simulink model "ControlSim"  (R2020b)
settings: Solver=VariableStepAuto  StartTime=0.0  StopTime=T  RelTol=1e-3
values from neighbouring files (symbols this model uses):
  condtheta = x0(3)    [MPCdefinition.m]
  condx = x0(1)    [MPCdefinition.m]
  condy = x0(2)    [MPCdefinition.m]
  dim_platform = 1.3    [MPCdefinition.m]
  k_obsx = 5    [MPCdefinition.m]
  k_obsy = 5    [MPCdefinition.m]
  omega_max_perc = 0.1    [MPCdefinition.m]
  omega_min_perc = -0.1    [MPCdefinition.m]
  omega_sat = 2    [MPCdefinition.m]
  slope_circ = 0.2    [MPCdefinition.m]
  v_max_perc = 0.5    [MPCdefinition.m]
  v_min_perc = -0.5    [MPCdefinition.m]
  v_square = 0.8    [MPCdefinition.m]
libraries: simulink x3, mpclib x1
settings Model: Creator=adelina  LastModifiedBy=adelina

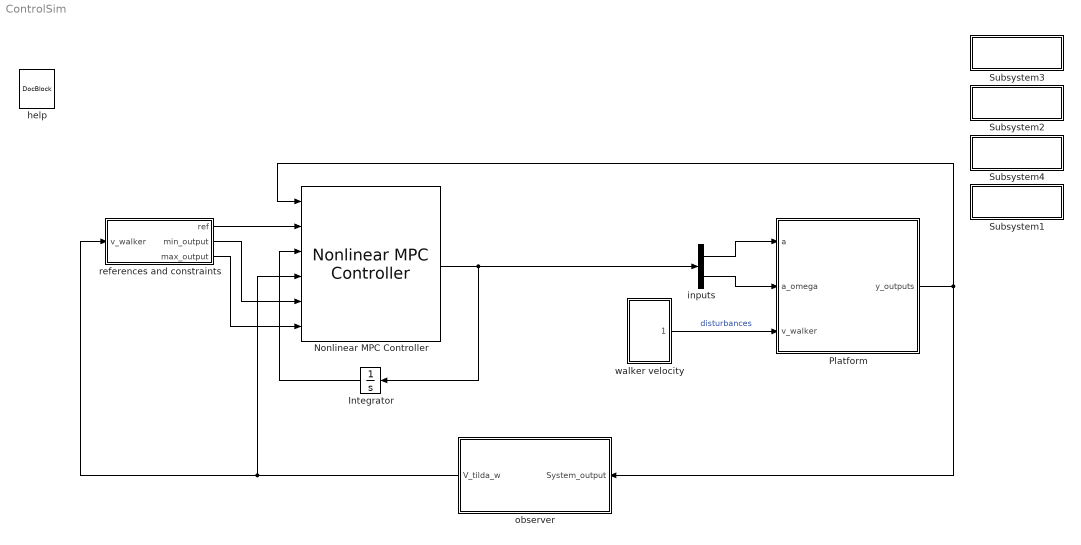
== system ControlSim ==
  Integrator : Integrator  InitialCondition=[0, 0]
  Nonlinear MPC Controller : mpclib/Nonlinear MPC Controller  SCDEnableBlockLinearizationSpecification=on  nlmpcobj=nlobj  UseObjectTs=on  UseMEX=off  md_enabled=on  mvtarget_enabled=off  param_enabled=off  cost_enabled=off  mvseq_enabled=off  stateseq_enabled=off  ovseq_enabled=off  slack_enabled=off  status_enabled=off  ov_min=on  ov_max=on  mv_min=off  mv_max=off  mvrate_min=off  mvrate_max=off  state_min=off  state_max=off  ov_weight=off  mv_weight=off  mvrate_weight=off  ecr_weight=off  nlp_initialize=off
  Platform : Subsystem
  Subsystem1 : Subsystem
      settings: OpenFcn=animation
      mask Display: disp('Animation')
  Subsystem2 : Subsystem
      settings: OpenFcn=plot_inputs
      mask Display: disp('plot inputs')
  Subsystem3 : Subsystem
      settings: OpenFcn=plot_states
      mask Display: disp('plot states')
  Subsystem4 : Subsystem
      settings: OpenFcn=plot_trajectory_frames
      mask Display: disp('plot trajectory')
  help : simulink/Model-Wide Utilities/DocBlock  DocumentType=Text
      content=|
      | 1. You may have errors running plot trajectory, this is due to the "for ... end" in the script, just ignore the error
      |
      | 2. To choose the trajectory go on the block "walker velocity"
  inputs : Demux  Outputs=2
  observer : Subsystem
  references and constraints : Subsystem
  walker velocity : Subsystem
  wires:
  inputs/2 -> Platform/2(a_omega)
  inputs/1 -> Platform/1(a)
  Integrator/1 -> Nonlinear MPC Controller/3
  references and constraints/1(ref) -> Nonlinear MPC Controller/2
  Platform/1(y_outputs) -> observer/1(System_output), Nonlinear MPC Controller/1
  walker velocity/1(v_walker) -> Platform/3(v_walker)  "disturbances"
  observer/1(V_tilda_w) -> Nonlinear MPC Controller/4, references and constraints/1(v_walker)
  references and constraints/2(min_output) -> Nonlinear MPC Controller/5
  references and constraints/3(max_output) -> Nonlinear MPC Controller/6
  Nonlinear MPC Controller/1 -> inputs/1, Integrator/1

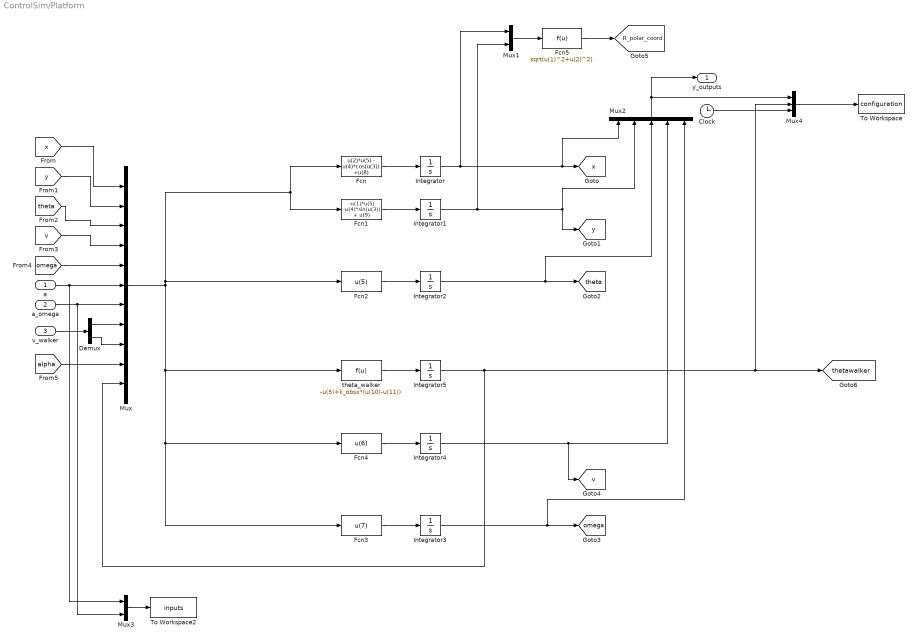
== system ControlSim/Platform ==
  a : Inport
  a_omega : Inport  Port=2
  v_walker : Inport  Port=3
  Clock : Clock
  Demux : Demux  Outputs=2
  Fcn : Fcn  Expr=u(2)*u(5) - u(4)*cos(u(3)) +u(8)
  Fcn1 : Fcn  Expr=-u(1)*u(5) -u(4)*sin(u(3)) + u(9)
  Fcn2 : Fcn  Expr=u(5)
  Fcn3 : Fcn  Expr=u(7)
  Fcn4 : Fcn  Expr=u(6)
  Fcn5 : Fcn  Expr=sqrt(u(1)^2+u(2)^2)
  Integrator : Integrator  InitialCondition=condx
  Integrator1 : Integrator  InitialCondition=condy
  Integrator2 : Integrator  InitialCondition=condtheta
  Integrator3 : Integrator
  Integrator4 : Integrator
  Integrator5 : Integrator  InitialCondition=condtheta
  Mux : Mux  Inputs=11
  Mux1 : Mux  Inputs=2
  Mux2 : Mux  Inputs=5
  Mux3 : Mux  Inputs=2
  Mux4 : Mux  Inputs=3
  To Workspace : ToWorkspace  VariableName=configuration  SaveFormat=Structure With Time  SampleTime=-1
  To Workspace2 : ToWorkspace  VariableName=inputs  SaveFormat=Structure With Time  SampleTime=-1
  theta_walker : Fcn  Expr=-u(5)+k_obsx*(u(10)-u(11))
  y_outputs : Outport
  tag scope: R_polar_coord=global, omega=global, theta=global, thetawalker=global, v=global, x=global, y=global
  wires:
  Fcn2/1 -> Integrator2/1
  Integrator2/1 -> [theta], Mux2/3
  Fcn1/1 -> Integrator1/1
  [y] -> Mux/2
  [x] -> Mux/1
  a/1 -> Mux3/1, Mux/6
  Integrator1/1 -> Mux1/2, [y], Mux2/2
  [theta] -> Mux/3
  Integrator/1 -> Mux1/1, Mux2/1, [x]
  Fcn/1 -> Integrator/1
  a_omega/1 -> Mux3/2, Mux/7
  Mux2/1 -> y_outputs/1, Mux4/1
  [v] -> Mux/4
  [omega] -> Mux/5
  Integrator3/1 -> Mux2/5, [omega]
  Fcn3/1 -> Integrator3/1
  Integrator4/1 -> [v], Mux2/4
  Fcn4/1 -> Integrator4/1
  Mux1/1 -> Fcn5/1
  Fcn5/1 -> [R_polar_coord]
  Mux3/1 -> To Workspace2/1
  Clock/1 -> Mux4/3
  Mux4/1 -> To Workspace/1
  v_walker/1 -> Demux/1
  Demux/1 -> Mux/8
  Demux/2 -> Mux/9
  [alpha] -> Mux/10
  Mux/1 -> Fcn1/1, Fcn/1, Fcn2/1, theta_walker/1, Fcn3/1, Fcn4/1
  theta_walker/1 -> Integrator5/1
  Integrator5/1 -> Mux/11, [thetawalker], Mux4/2

== system ControlSim/Subsystem1 ==

== system ControlSim/Subsystem2 ==

== system ControlSim/Subsystem3 ==

== system ControlSim/Subsystem4 ==

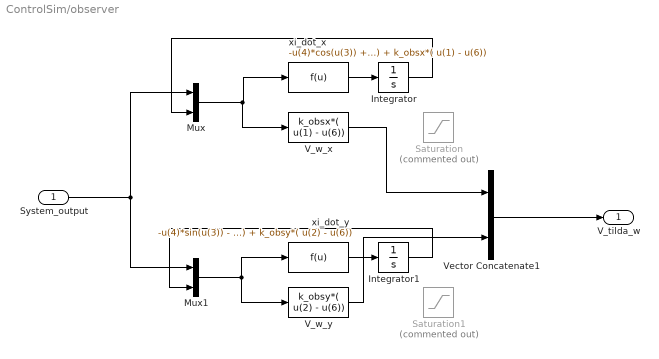
== system ControlSim/observer ==
  System_output : Inport
  Integrator : Integrator  InitialCondition=condx
  Integrator1 : Integrator  InitialCondition=condy
  Mux : Mux  Inputs=2
  Mux1 : Mux  Inputs=2
  Saturation : Saturate  Commented=on
  Saturation1 : Saturate  Commented=on
  V_w_x : Fcn  Expr=k_obsx*( u(1) - u(6))
  V_w_y : Fcn  Expr=k_obsy*( u(2) - u(6))
  Vector Concatenate1 : Concatenate  Mode=Multidimensional array  ConcatenateDimension=2
  xi_dot_x : Fcn  Expr=-u(4)*cos(u(3)) + u(2)*u(5) + k_obsx*( u(1) - u(6))
  xi_dot_y : Fcn  Expr=-u(4)*sin(u(3)) - u(1)*u(5) + k_obsy*( u(2) - u(6))
  V_tilda_w : Outport
  wires:
  Mux/1 -> V_w_x/1, xi_dot_x/1
  Mux1/1 -> V_w_y/1, xi_dot_y/1
  System_output/1 -> Mux/1, Mux1/1
  Vector Concatenate1/1 -> V_tilda_w/1
  xi_dot_x/1 -> Integrator/1
  Integrator/1 -> Mux/2
  xi_dot_y/1 -> Integrator1/1
  Integrator1/1 -> Mux1/2
  V_w_y/1 -> Vector Concatenate1/2
  V_w_x/1 -> Vector Concatenate1/1

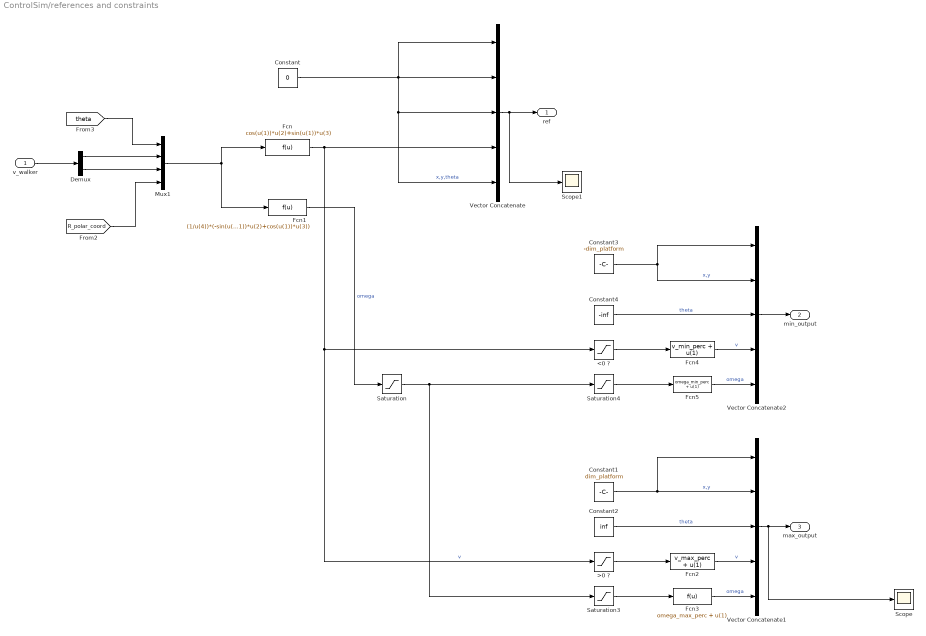
== system ControlSim/references and constraints ==
  v_walker : Inport
  <0 ? : Saturate  UpperLimit=0  LowerLimit=-inf
  >0 ? : Saturate  UpperLimit=inf  LowerLimit=0
  Constant : Constant  Value=0
  Constant1 : Constant  Value=dim_platform
  Constant2 : Constant  Value=inf
  Constant3 : Constant  Value=-dim_platform
  Constant4 : Constant  Value=-inf
  Demux : Demux  Outputs=2
  Fcn : Fcn  Expr=cos(u(1))*u(2)+sin(u(1))*u(3)
  Fcn1 : Fcn  Expr=(1/u(4))*(-sin(u(1))*u(2)+cos(u(1))*u(3))
  Fcn2 : Fcn  Expr=v_max_perc + u(1)
  Fcn3 : Fcn  Expr=omega_max_perc + u(1)
  Fcn4 : Fcn  Expr=v_min_perc + u(1)
  Fcn5 : Fcn  Expr=omega_min_perc + u(1)
  Mux1 : Mux
  Saturation : Saturate  UpperLimit=omega_sat  LowerLimit=-omega_sat
  Saturation3 : Saturate  UpperLimit=inf  LowerLimit=0
  Saturation4 : Saturate  UpperLimit=0  LowerLimit=-inf
  Scope : Scope
  Scope1 : Scope
  Vector Concatenate : Concatenate  NumInputs=5  Mode=Multidimensional array  ConcatenateDimension=2
  Vector Concatenate1 : Concatenate  NumInputs=5  Mode=Multidimensional array  ConcatenateDimension=2
  Vector Concatenate2 : Concatenate  NumInputs=5  Mode=Multidimensional array  ConcatenateDimension=2
  ref : Outport
  min_output : Outport  Port=2
  max_output : Outport  Port=3
  wires:
  Constant/1 -> Vector Concatenate/1, Vector Concatenate/5, Vector Concatenate/3, Vector Concatenate/2  "x,y,theta"
  Vector Concatenate/1 -> Scope1/1, ref/1
  [R_polar_coord] -> Mux1/4
  [theta] -> Mux1/1
  Demux/1 -> Mux1/2
  Demux/2 -> Mux1/3
  Fcn1/1 -> Saturation/1  "omega"
  Fcn2/1 -> Vector Concatenate1/4  "v"
  Constant1/1 -> Vector Concatenate1/1, Vector Concatenate1/2  "x,y"
  Mux1/1 -> Fcn/1, Fcn1/1
  Fcn3/1 -> Vector Concatenate1/5  "omega"
  Constant2/1 -> Vector Concatenate1/3  "theta"
  >0 ?/1 -> Fcn2/1
  Saturation3/1 -> Fcn3/1
  Fcn5/1 -> Vector Concatenate2/5  "omega"
  Constant4/1 -> Vector Concatenate2/3  "theta"
  Saturation/1 -> Saturation3/1, Saturation4/1
  Fcn/1 -> Vector Concatenate/4, >0 ?/1, <0 ?/1  "v"
  Fcn4/1 -> Vector Concatenate2/4  "v"
  Saturation4/1 -> Fcn5/1
  <0 ?/1 -> Fcn4/1
  Constant3/1 -> Vector Concatenate2/2, Vector Concatenate2/1  "x,y"
  Vector Concatenate2/1 -> min_output/1
  Vector Concatenate1/1 -> Scope/1, max_output/1
  v_walker/1 -> Demux/1

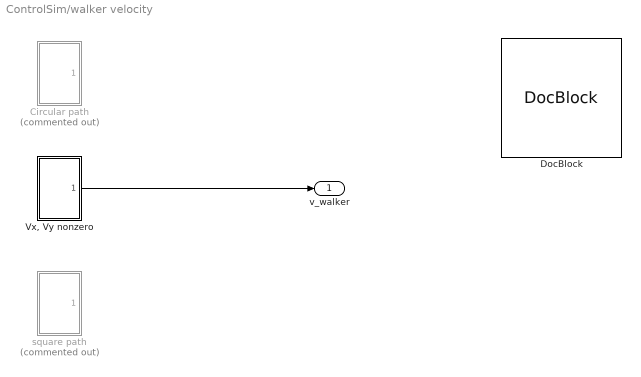
== system ControlSim/walker velocity ==
  Circular path : Subsystem  Commented=on
  DocBlock : simulink/Model-Wide Utilities/DocBlock  DocumentType=Text
      content=|
      | Choose one of the trajectory by uncommenting and connecting with the output
  "Vx, Vy nonzero" : Subsystem
  square path : Subsystem  Commented=on
  v_walker : Outport
  wires:
  "Vx, Vy nonzero"/1(v_walker) -> v_walker/1

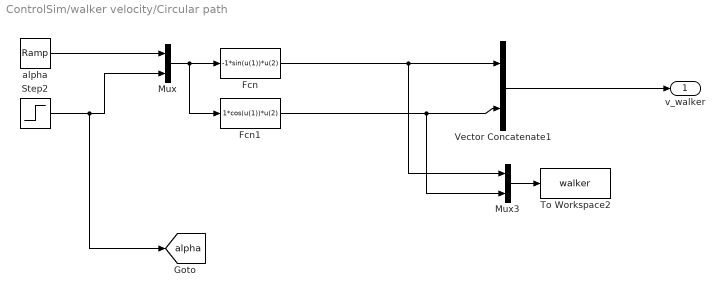
== system ControlSim/walker velocity/Circular path ==
  Fcn : Fcn  Expr=-1*sin(u(1))*u(2)
  Fcn1 : Fcn  Expr=1*cos(u(1))*u(2)
  Mux : Mux  Inputs=2
  Mux3 : Mux  Inputs=2
  Step2 : Step  After=slope_circ  SampleTime=0
  To Workspace2 : ToWorkspace  VariableName=walker  SaveFormat=Structure With Time  SampleTime=-1
  Vector Concatenate1 : Concatenate  Mode=Multidimensional array  ConcatenateDimension=2
  alpha : simulink/Sources/Ramp  slope=slope_circ  start=1  InitialOutput=0
  v_walker : Outport
  tag scope: alpha=global
  wires:
  alpha/1 -> Mux/1
  Fcn1/1 -> Vector Concatenate1/2, Mux3/2
  Fcn/1 -> Mux3/1, Vector Concatenate1/1
  Vector Concatenate1/1 -> v_walker/1
  Mux3/1 -> To Workspace2/1
  Mux/1 -> Fcn1/1, Fcn/1
  Step2/1 -> [alpha], Mux/2

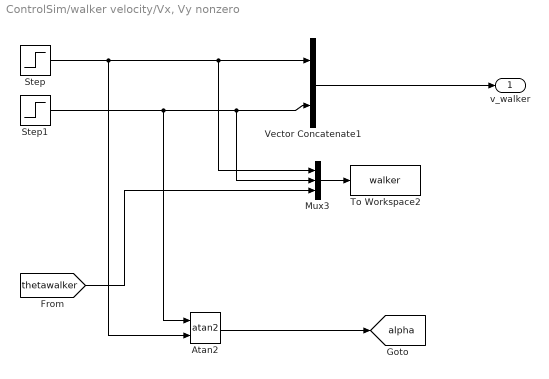
== system ControlSim/walker velocity/Vx, Vy nonzero ==
  Atan2 : Trigonometry  Operator=atan2
  Mux3 : Mux  Inputs=3
  Step : Step  Time=12  After=0.7  SampleTime=0
  Step1 : Step  Time=2  After=0.4  SampleTime=0
  To Workspace2 : ToWorkspace  VariableName=walker  SaveFormat=Structure With Time  SampleTime=-1
  Vector Concatenate1 : Concatenate  Mode=Multidimensional array  ConcatenateDimension=2
  v_walker : Outport
  tag scope: alpha=global
  wires:
  Vector Concatenate1/1 -> v_walker/1
  Mux3/1 -> To Workspace2/1
  Step/1 -> Atan2/2, Mux3/1, Vector Concatenate1/1
  Step1/1 -> Atan2/1, Vector Concatenate1/2, Mux3/2
  [thetawalker] -> Mux3/3
  Atan2/1 -> [alpha]

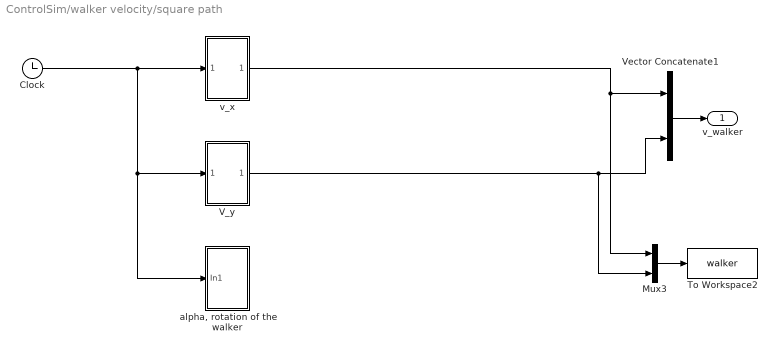
== system ControlSim/walker velocity/square path ==
  Clock : Clock
  Mux3 : Mux  Inputs=2
  To Workspace2 : ToWorkspace  VariableName=walker  SaveFormat=Structure With Time  SampleTime=-1
  V_y : Subsystem
  Vector Concatenate1 : Concatenate  Mode=Multidimensional array  ConcatenateDimension=2
  "alpha, rotation of the walker" : Subsystem
  v_x : Subsystem
  v_walker : Outport
  wires:
  Vector Concatenate1/1 -> v_walker/1
  Mux3/1 -> To Workspace2/1
  Clock/1 -> v_x/1(In1), "alpha, rotation of the walker"/1(In1), V_y/1(In1)
  V_y/1(Out1) -> Mux3/2, Vector Concatenate1/2
  v_x/1(Out1) -> Mux3/1, Vector Concatenate1/1

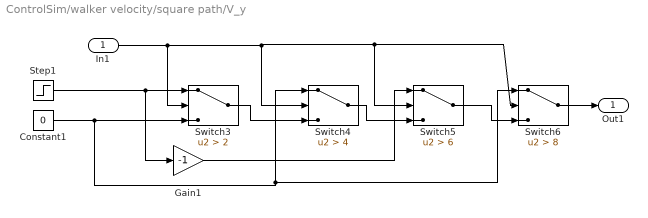
== system ControlSim/walker velocity/square path/V_y ==
  In1 : Inport
  Constant1 : Constant  Value=0
  Gain1 : Gain  Gain=-1
  Step1 : Step  Time=0  After=v_square  SampleTime=0
  Switch3 : Switch  Criteria=u2 > Threshold  Threshold=2
  Switch4 : Switch  Criteria=u2 > Threshold  Threshold=4
  Switch5 : Switch  Criteria=u2 > Threshold  Threshold=6
  Switch6 : Switch  Criteria=u2 > Threshold  Threshold=8
  Out1 : Outport
  wires:
  Step1/1 -> Gain1/1, Switch3/1
  Switch6/1 -> Out1/1
  In1/1 -> Switch3/2, Switch5/2, Switch6/2, Switch4/2
  Switch5/1 -> Switch6/3
  Switch3/1 -> Switch4/3
  Constant1/1 -> Switch6/1, Switch4/1, Switch3/3
  Switch4/1 -> Switch5/3
  Gain1/1 -> Switch5/1

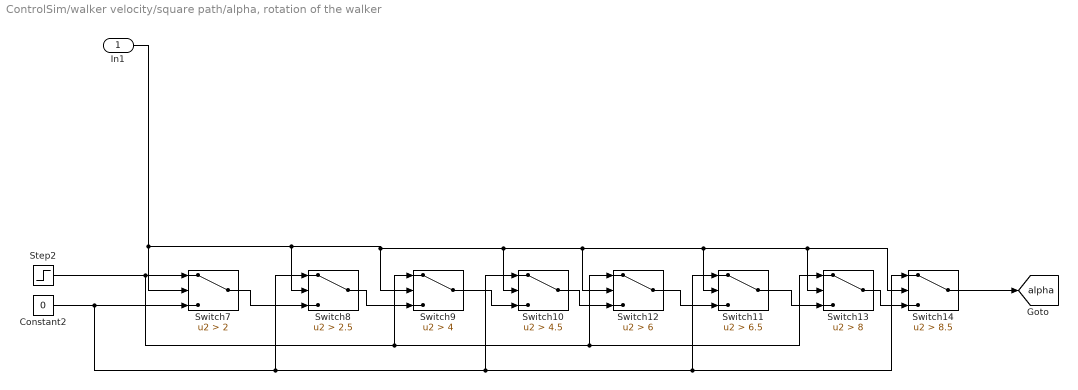
== system ControlSim/walker velocity/square path/alpha, rotation of the walker ==
  In1 : Inport
  Constant2 : Constant  Value=0
  Step2 : Step  Time=0  After=pi  SampleTime=0
  Switch10 : Switch  Criteria=u2 > Threshold  Threshold=4.5
  Switch11 : Switch  Criteria=u2 > Threshold  Threshold=6.5
  Switch12 : Switch  Criteria=u2 > Threshold  Threshold=6
  Switch13 : Switch  Criteria=u2 > Threshold  Threshold=8
  Switch14 : Switch  Criteria=u2 > Threshold  Threshold=8.5
  Switch7 : Switch  Criteria=u2 > Threshold  Threshold=2
  Switch8 : Switch  Criteria=u2 > Threshold  Threshold=2.5
  Switch9 : Switch  Criteria=u2 > Threshold  Threshold=4
  tag scope: alpha=global
  wires:
  Switch11/1 -> Switch13/3
  Switch13/1 -> Switch14/3
  Switch14/1 -> [alpha]
  In1/1 -> Switch8/2, Switch12/2, Switch14/2, Switch13/2, Switch11/2, Switch10/2, Switch9/2, Switch7/2
  Switch9/1 -> Switch10/3
  Switch8/1 -> Switch9/3
  Switch10/1 -> Switch12/3
  Switch7/1 -> Switch8/3
  Step2/1 -> Switch9/1, Switch13/1, Switch12/1, Switch7/1
  Constant2/1 -> Switch8/1, Switch10/1, Switch11/1, Switch14/1, Switch7/3
  Switch12/1 -> Switch11/3

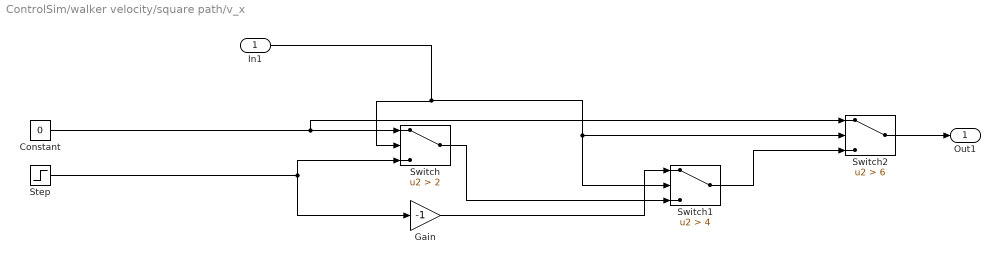
== system ControlSim/walker velocity/square path/v_x ==
  In1 : Inport
  Constant : Constant  Value=0
  Gain : Gain  Gain=-1
  Step : Step  Time=0  After=v_square  SampleTime=0
  Switch : Switch  Criteria=u2 > Threshold  Threshold=2
  Switch1 : Switch  Criteria=u2 > Threshold  Threshold=4
  Switch2 : Switch  Criteria=u2 > Threshold  Threshold=6
  Out1 : Outport
  wires:
  Switch1/1 -> Switch2/3
  In1/1 -> Switch/2, Switch1/2, Switch2/2
  Gain/1 -> Switch1/1
  Switch/1 -> Switch1/3
  Step/1 -> Gain/1, Switch/3
  Constant/1 -> Switch2/1, Switch/1
  Switch2/1 -> Out1/1
